simulink model "exampleWorkingTime"  (R2013b)
settings: Solver=ode45  StartTime=0.0  StopTime=30  RelTol=1e-3
libraries: carnot x1
settings Model: Creator=drhf  LastModifiedBy=drhf
settings OptimizationCC: InlineParams=on

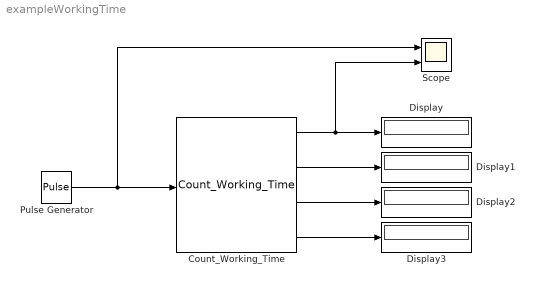
== system exampleWorkingTime ==
  Count_Working_Time : carnot/Toolbox/Count_Working_Time
  Display{,1..3} (4 alike) : Display
  Pulse Generator : DiscretePulseGenerator  PulseType=Time based  Period=10  PulseWidth=10  PhaseDelay=1
  Scope : Scope  NumInputPorts=2
      settings: YMin=-5~-5  YMax=5~5
  wires:
  Pulse Generator/1 -> Scope/1, Count_Working_Time/1
  Count_Working_Time/1 -> Scope/2, Display/1
  Count_Working_Time/2 -> Display1/1
  Count_Working_Time/3 -> Display2/1
  Count_Working_Time/4 -> Display3/1
